simulink model "feedbacksystem"  (Simulink 6.0)
settings: Solver=ode5  StartTime=0.0  StopTime=10.0  RelTol=1e-3
settings Model: Creator=The MathWorks Inc.  LastModifiedBy=batserve  ExtModeTrigMode=oneshot  ExtModeArmWhenConnect=off  ExtModeAutoUpdateStatusClock=off
settings DataIOCC: LimitDataPoints=off
settings OptimizationCC: BlockReduction=off  BooleanDataType=off
settings DebuggingCC: CheckExecutionContextPreStartOutputMsg=on  CheckExecutionContextRuntimeOutputMsg=on  SolverPrmCheckMsg=none
settings HardwareCC: TargetUnknown=on

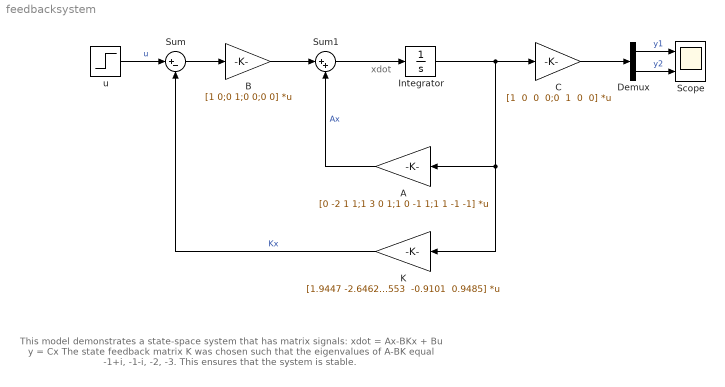
== system feedbacksystem ==
  note: xdot
  note: This model demonstrates a state-space system that has matrix signals:
      |
      | xdot = Ax-BKx + Bu
      | y = Cx
      |
      | The state feedback matrix K was chosen such that the eigenvalues of
      | A-BK equal -1+i, -1-i, -2, -3. This ensures that the system is stable.
  A : Gain  Orientation=left  Gain=[0 -2 1 1;1 3 0 1;1 0 -1 1;1 1 -1 -1]  Multiplication=Matrix(K*u)  SaturateOnIntegerOverflow=on
  B : Gain  Gain=[1 0;0 1;0 0;0 0]  Multiplication=Matrix(K*u)  SaturateOnIntegerOverflow=on
  C : Gain  Gain="[1  0  0  0;0  1  0  0]"  Multiplication=Matrix(K*u)  SaturateOnIntegerOverflow=on
  Demux : Demux  Outputs=2
  Integrator : Integrator
  K : Gain  Orientation=left  Gain="[1.9447 -2.6462 1.6214  0.7910;0.5320  6.0553  -0.9101  0.9485]"  Multiplication=Matrix(K*u)  SaturateOnIntegerOverflow=on
  Scope : Scope  NumInputPorts=2
      settings: TimeRange=10  YMin=0~0  YMax=0.8~0.8
  Sum : Sum  Inputs=|+-  SaturateOnIntegerOverflow=on  InputSameDT=on
  Sum1 : Sum  Inputs=|++  SaturateOnIntegerOverflow=on  InputSameDT=on
  u : Step  Time=[0 0]'  SampleTime=0  VectorParams1D=off
  wires:
  u/1 -> Sum/1  "u"
  Sum/1 -> B/1
  Integrator/1 -> C/1, K/1, A/1
  Sum1/1 -> Integrator/1
  C/1 -> Demux/1
  Demux/1 -> Scope/1  "y1"
  Demux/2 -> Scope/2  "y2"
  B/1 -> Sum1/1
  K/1 -> Sum/2  "Kx"
  A/1 -> Sum1/2  "Ax"
